simulink model "MSD_PID_SMC_v01"  (R2022b)
settings: Solver=ode45  StartTime=0.0  StopTime=10  FixedStep=Ts  MaxStep=1e-2  RelTol=1e-3
values from neighbouring files (symbols this model uses):
  c = zeta*ccr    [Sphere2.m]
  k = 1e3    (= 1000)    [Sphere2.m]
  m = 10e-3    (= 0.01)    [Sphere2.m]
undefined symbols (not defined in the file or in its folder): Epsilon, Kd, Ki, Kp, KSMC, Lambda
settings Model: Creator=ababaei  LastModifiedBy=ababaei
settings SolverCC: AlgebraicLoopSolver=LineSearch
settings DataIOCC: ExternalInput=[spg.setpoint.t, dist.Fz_IH]
settings DebuggingCC: ArtificialAlgebraicLoopMsg=none  MaxConsecutiveZCsMsg=warning  MultiTaskDSMMsg=warning  MultiTaskCondExecSysMsg=warning  MultiTaskRateTransMsg=warning  ParameterDowncastMsg=warning  ParameterOverflowMsg=warning  UnconnectedInputMsg=warning  UnconnectedOutputMsg=warning  UnconnectedLineMsg=warning  FrameProcessingCompatibilityMsg=warning  ModelReferenceExtraNoncontSigs=warning  NonCurrentReleaseOperatingPointMsg=warning  SFUnexpectedBacktrackingDiag=warning  SFNoUnconditionalDefaultTransitionDiag=warning  SFOutputUsedAsStateInMooreChartDiag=warning  SFMachineParentedDataDiag=warning  ArithmeticOperatorsInVariantConditions=warning
settings ModelReferenceCC: EnableRefExpFcnMdlSchedulingChecks=on
settings SFSimCC: SimUseLocalCustomCode=off  CustomCodeUndefinedFunction=UseInterfaceOnly
settings RTWCC: RTWUseLocalCustomCode=off
settings CodeAppCC: StateflowObjectComments=on

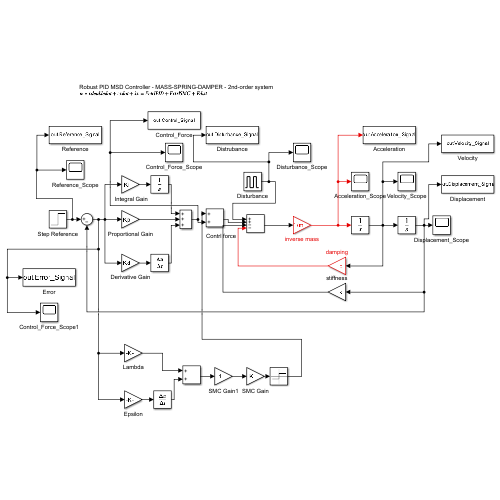
[thumbnail: Simulink's stored preview of the top-level diagram]
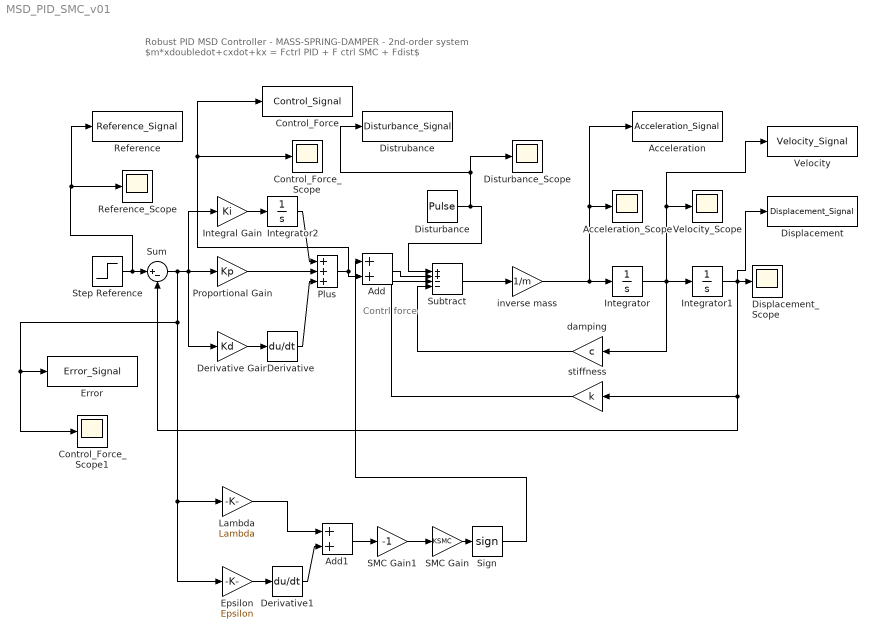
== system MSD_PID_SMC_v01 ==
  note: Robust PID MSD Controller - MASS-SPRING-DAMPER - 2nd-order system
      | $m*xdoubledot+cxdot+kx = Fctrl PID + F ctrl SMC + Fdist$
  note: Contrl force
  " Integral Gain" : Gain  Gain=Ki
  Acceleration : ToWorkspace  VariableName=Acceleration_Signal  SaveFormat=Timeseries  SampleTime=-1
  Acceleration_Scope : Scope
  Add : Sum
  Add1 : Sum
  Control_Force : ToWorkspace  VariableName=Control_Signal  SaveFormat=Timeseries  SampleTime=-1
  Control_Force_Scope : Scope
  Control_Force_Scope1 : Scope
  Derivative : Derivative
  Derivative Gain : Gain  Gain=Kd
  Derivative1 : Derivative
  Displacement : ToWorkspace  VariableName=Displacement_Signal  SaveFormat=Timeseries  SampleTime=-1
  Displacement_Scope : Scope
  Distrubance : ToWorkspace  VariableName=Disturbance_Signal  SaveFormat=Timeseries  SampleTime=-1
  Disturbance : DiscretePulseGenerator  PulseType=Time based  Amplitude=0.5  Period=20  PulseWidth=2
  Disturbance_Scope : Scope
  Epsilon : Gain  Gain=Epsilon
  Error : ToWorkspace  VariableName=Error_Signal  SaveFormat=Timeseries  SampleTime=-1
  Integrator : Integrator
  Integrator1 : Integrator
  Integrator2 : Integrator
  Lambda : Gain  Gain=Lambda
  Plus : Sum  Inputs=+++
  Proportional Gain : Gain  Gain=Kp
  Reference : ToWorkspace  VariableName=Reference_Signal  SaveFormat=Timeseries  SampleTime=-1
  Reference_Scope : Scope
  SMC Gain : Gain  Gain=KSMC
  SMC Gain1 : Gain  Gain=-1
  Sign : Signum
  Step Reference : Step  Time=0  SampleTime=0
  Subtract : Sum  Inputs=++--
  Sum : Sum  Inputs=|+-
  Velocity : ToWorkspace  VariableName=Velocity_Signal  SaveFormat=Timeseries  SampleTime=-1
  Velocity_Scope : Scope
  damping : Gain  Gain=c
  inverse mass : Gain  Gain=1/m
  stiffness : Gain  Gain=k
  wires:
  Subtract/1 -> inverse mass/1
  inverse mass/1 -> Acceleration/1, Acceleration_Scope/1, Integrator/1
  damping/1 -> Subtract/4
  Integrator/1 -> damping/1, Velocity/1, Velocity_Scope/1, Integrator1/1
  stiffness/1 -> Subtract/3
  Integrator1/1 -> Displacement/1, stiffness/1, Sum/2, Displacement_Scope/1
  Disturbance/1 -> Subtract/1, Distrubance/1, Disturbance_Scope/1
  Derivative Gain/1 -> Derivative/1
  " Integral Gain"/1 -> Integrator2/1
  Step Reference/1 -> Reference/1, Reference_Scope/1, Sum/1
  Derivative/1 -> Plus/3
  Proportional Gain/1 -> Plus/2
  Integrator2/1 -> Plus/1
  Plus/1 -> Add/2, Control_Force/1, Control_Force_Scope/1
  Add/1 -> Subtract/2
  Sum/1 -> Epsilon/1, Lambda/1, Control_Force_Scope1/1, Error/1, Derivative Gain/1, " Integral Gain"/1, Proportional Gain/1
  Epsilon/1 -> Derivative1/1
  Lambda/1 -> Add1/1
  Derivative1/1 -> Add1/2
  Add1/1 -> SMC Gain1/1
  SMC Gain/1 -> Sign/1
  SMC Gain1/1 -> SMC Gain/1
  Sign/1 -> Add/1
